simulink model "MinSeg_sim_LQR"  (R2024b)
settings: Solver=ode4  StartTime=0.0  StopTime=4  FixedStep=0.0001  RelTol=1e-3
values from neighbouring files (symbols this model uses):
  c = 0.5    [parameters.m]
  d = 0.5    [parameters.m]
  eta = 0.9    [parameters.m]
  g = 9.81    [parameters.m]
  I = M/12*(t^2 + b^2) + M*l^2    (= 0.00128463833333)    [parameters.m]
  J = 1/2*m*r^2    (= 2.7104e-05)    [parameters.m]
  K = lqr(sys_MS, Q_lqr, R_lqr)    [main.m]
  Km = 0.05    [parameters.m]
  L = 2.6e-3    (= 0.0026)    [parameters.m]    (also in pole_placement_Luenberger.m = place(A', C', desired_poles)')
  l = 0.06    [parameters.m]
  M = 0.3303 - 2*m    (= 0.2743)    [parameters.m]
  m = 0.028    [parameters.m]
  N = 50    [parameters.m]
  R = 0.5    [parameters.m]
  r = 0.044    [parameters.m]
undefined symbols (not defined in the file or in its folder): init_dq, init_q, tau_m, tau_max, theta_ref, U_max
settings Model: Creator=albin  LastModifiedBy=albin
settings DataIOCC: ExternalInput=[t, 6, 6]  ReturnWorkspaceOutputs=off

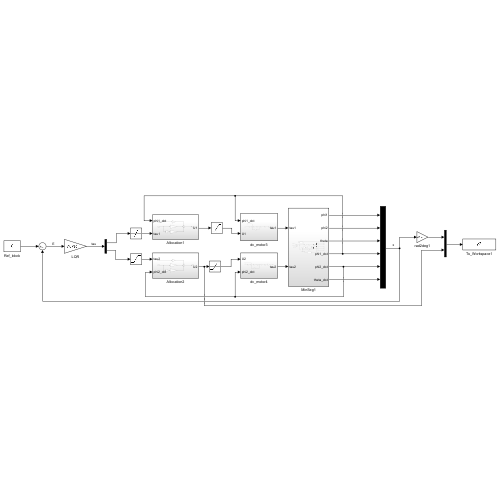
[thumbnail: Simulink's stored preview of the top-level diagram]
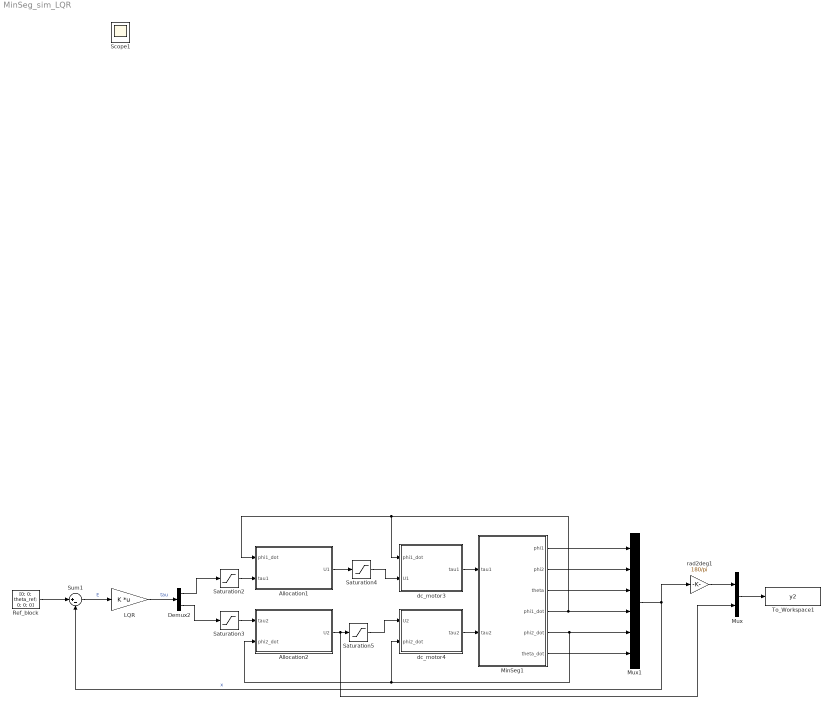
== system MinSeg_sim_LQR ==
  Allocation1 : Subsystem
  Allocation2 : Subsystem
  Demux2 : Demux  Outputs=2
  LQR : Gain  Gain=K  Multiplication=Matrix(K*u) (u vector)
  MinSeg1 : Subsystem
  Mux : Mux  Inputs=2
  Mux1 : Mux  Inputs=6
  Ref_block : Constant  Value=[0; 0; theta_ref; 0; 0; 0]
  Saturation2 : Saturate  UpperLimit=tau_max  LowerLimit=-tau_max
  Saturation3 : Saturate  UpperLimit=0.05  LowerLimit=-0.05
  Saturation4 : Saturate  UpperLimit=U_max  LowerLimit=-U_max
  Saturation5 : Saturate  UpperLimit=U_max  LowerLimit=-U_max
  Sum1 : Sum  Inputs=|+-
  To_Workspace1 : ToWorkspace  VariableName=y2  SaveFormat=Timeseries  SampleTime=-1
  dc_motor3 : Subsystem
  dc_motor4 : Subsystem
  rad2deg1 : Gain  Gain=180/pi
  Scope1 : Scope
  wires:
  Allocation2/1(U2) -> Mux/2, Saturation5/1
  dc_motor4/1(tau2) -> MinSeg1/2(tau2)
  Saturation3/1 -> Allocation2/1(tau2)
  dc_motor3/1(tau1) -> MinSeg1/1(tau1)
  LQR/1 -> Demux2/1  "tau"
  Allocation1/1(U1) -> Saturation4/1
  MinSeg1/5(phi2_dot) -> Mux1/5, dc_motor4/2(phi2_dot), Allocation2/2(phi2_dot)
  Sum1/1 -> LQR/1  "E"
  Demux2/1 -> Saturation2/1
  MinSeg1/4(phi1_dot) -> Allocation1/1(phi1_dot), dc_motor3/1(phi1_dot), Mux1/4
  Mux1/1 -> rad2deg1/1, Sum1/2  "x"
  Saturation2/1 -> Allocation1/2(tau1)
  MinSeg1/1(phi1) -> Mux1/1
  Ref_block/1 -> Sum1/1
  MinSeg1/6(theta_dot) -> Mux1/6
  MinSeg1/2(phi2) -> Mux1/2
  Saturation4/1 -> dc_motor3/2(U1)
  Saturation5/1 -> dc_motor4/1(U2)
  MinSeg1/3(theta) -> Mux1/3
  Demux2/2 -> Saturation3/1
  Mux/1 -> To_Workspace1/1
  rad2deg1/1 -> Mux/1

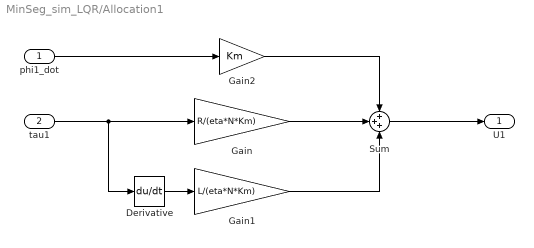
== system MinSeg_sim_LQR/Allocation1 ==
  phi1_dot : Inport
  tau1 : Inport  Port=2
  Derivative : Derivative
  Gain : Gain  Gain=R/(eta*N*Km)
  Gain1 : Gain  Gain=L/(eta*N*Km)
  Gain2 : Gain  Gain=Km
  Sum : Sum  Inputs=+++
  U1 : Outport
  wires:
  Gain1/1 -> Sum/3
  tau1/1 -> Derivative/1, Gain/1
  Gain/1 -> Sum/2
  Derivative/1 -> Gain1/1
  Sum/1 -> U1/1
  phi1_dot/1 -> Gain2/1
  Gain2/1 -> Sum/1

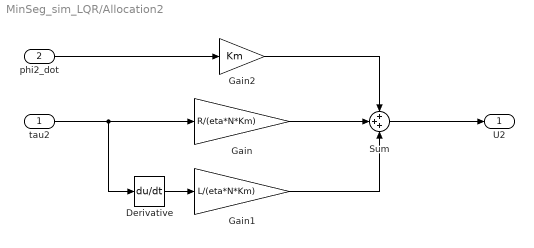
== system MinSeg_sim_LQR/Allocation2 ==
  tau2 : Inport
  phi2_dot : Inport  Port=2
  Derivative : Derivative
  Gain : Gain  Gain=R/(eta*N*Km)
  Gain1 : Gain  Gain=L/(eta*N*Km)
  Gain2 : Gain  Gain=Km
  Sum : Sum  Inputs=+++
  U2 : Outport
  wires:
  Gain1/1 -> Sum/3
  tau2/1 -> Derivative/1, Gain/1
  Gain/1 -> Sum/2
  Derivative/1 -> Gain1/1
  Sum/1 -> U2/1
  phi2_dot/1 -> Gain2/1
  Gain2/1 -> Sum/1

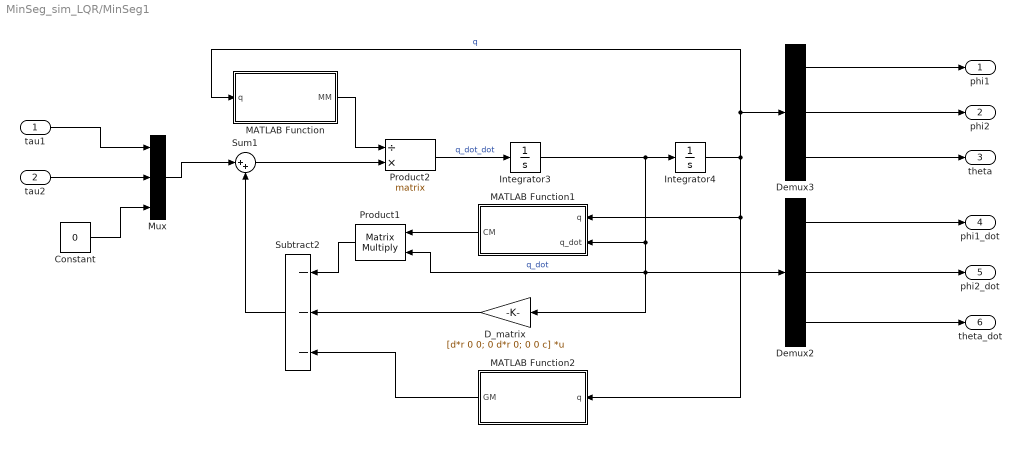
== system MinSeg_sim_LQR/MinSeg1 ==
  tau1 : Inport
  tau2 : Inport  Port=2
  Constant : Constant  Value=0
  D_matrix : Gain  Gain=[d*r 0 0; 0 d*r 0; 0 0 c]  Multiplication=Matrix(K*u)
  Demux2 : Demux  Outputs=3
  Demux3 : Demux  Outputs=3
  Integrator3 : Integrator  InitialCondition=init_dq
  Integrator4 : Integrator  InitialCondition=init_q
  MATLAB Function : MATLAB Function  TreatAsAtomicUnit=on
  MATLAB Function1 : MATLAB Function  TreatAsAtomicUnit=on
  MATLAB Function2 : MATLAB Function  TreatAsAtomicUnit=on
  Mux : Mux  Inputs=3
  Product1 : Product  Multiplication=Matrix(*)
  Product2 : Product  Inputs=/*  Multiplication=Matrix(*)
  Subtract2 : Sum  Inputs=---
  Sum1 : Sum  Inputs=|++
  phi1 : Outport
  phi2 : Outport  Port=2
  theta : Outport  Port=3
  phi1_dot : Outport  Port=4
  phi2_dot : Outport  Port=5
  theta_dot : Outport  Port=6
  wires:
  Product2/1 -> Integrator3/1  "q_dot_dot"
  Mux/1 -> Sum1/1
  Constant/1 -> Mux/3
  Integrator4/1 -> MATLAB Function2/1(q), MATLAB Function1/1(q), Demux3/1, MATLAB Function/1(q)  "q"
  Demux3/2 -> phi2/1
  Demux2/1 -> phi1_dot/1
  MATLAB Function/1(MM) -> Product2/1
  Demux3/1 -> phi1/1
  Integrator3/1 -> MATLAB Function1/2(q_dot), D_matrix/1, Product1/2, Demux2/1, Integrator4/1  "q_dot"
  MATLAB Function2/1(GM) -> Subtract2/3
  Subtract2/1 -> Sum1/2
  MATLAB Function1/1(CM) -> Product1/1
  Product1/1 -> Subtract2/1
  Demux2/3 -> theta_dot/1
  Demux2/2 -> phi2_dot/1
  Demux3/3 -> theta/1
  Sum1/1 -> Product2/2
  D_matrix/1 -> Subtract2/2
  tau1/1 -> Mux/1
  tau2/1 -> Mux/2

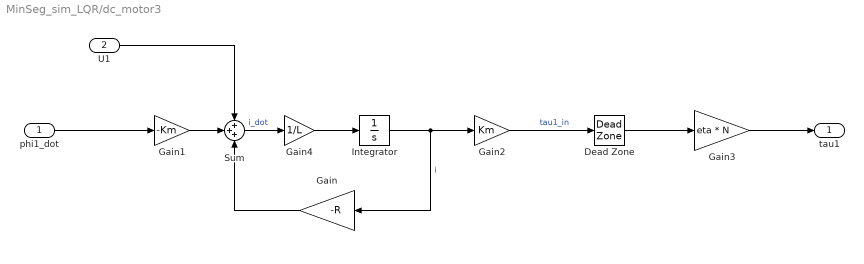
== system MinSeg_sim_LQR/dc_motor3 ==
  phi1_dot : Inport
  U1 : Inport  Port=2
  Dead Zone : DeadZone  LowerValue=-tau_m  UpperValue=tau_m
  Gain : Gain  Gain=-R
  Gain1 : Gain  Gain=-Km
  Gain2 : Gain  Gain=Km
  Gain3 : Gain  Gain=eta * N
  Gain4 : Gain  Gain=1/L
  Integrator : Integrator
  Sum : Sum  Inputs=+++
  tau1 : Outport
  wires:
  Gain2/1 -> Dead Zone/1  "tau1_in"
  Integrator/1 -> Gain/1, Gain2/1  "i"
  Gain3/1 -> tau1/1
  Gain1/1 -> Sum/2
  Gain/1 -> Sum/3
  phi1_dot/1 -> Gain1/1
  Sum/1 -> Gain4/1  "i_dot"
  Gain4/1 -> Integrator/1
  U1/1 -> Sum/1
  Dead Zone/1 -> Gain3/1

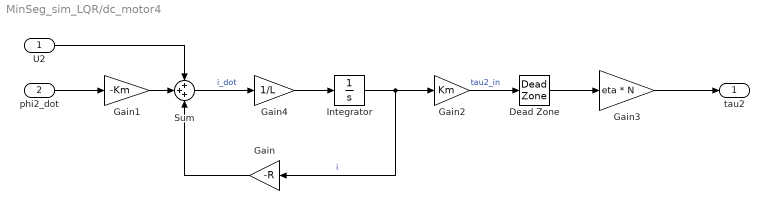
== system MinSeg_sim_LQR/dc_motor4 ==
  U2 : Inport
  phi2_dot : Inport  Port=2
  Dead Zone : DeadZone  LowerValue=-tau_m  UpperValue=tau_m
  Gain : Gain  Gain=-R
  Gain1 : Gain  Gain=-Km
  Gain2 : Gain  Gain=Km
  Gain3 : Gain  Gain=eta * N
  Gain4 : Gain  Gain=1/L
  Integrator : Integrator
  Sum : Sum  Inputs=+++
  tau2 : Outport
  wires:
  Gain2/1 -> Dead Zone/1  "tau2_in"
  Integrator/1 -> Gain/1, Gain2/1  "i"
  Gain3/1 -> tau2/1
  U2/1 -> Sum/1
  Gain1/1 -> Sum/2
  Sum/1 -> Gain4/1  "i_dot"
  phi2_dot/1 -> Gain1/1
  Gain/1 -> Sum/3
  Dead Zone/1 -> Gain3/1
  Gain4/1 -> Integrator/1

== matlab function MinSeg_sim_LQR/MinSeg1/MATLAB Function ==
  data: q input; MM output; r parameter; m parameter; M parameter; l parameter; I parameter; J parameter
function MM = M_matrix(q, r, m, M, l, I, J)
    % initialize
    MM = zeros(3,3);
    
    % extract theta from q
    theta = q(3);

    % Calculate the elements of the M(q) matrix
    MM(1,1) = r^2*(1/4*M + m) + J;
    MM(1,2) = 1/4*M*r^2;
    MM(1,3) = r^2*(1/2*M + m) + J + 1/2*M*l*r*cos(theta);
    MM(2,1) = 1/4*M*r^2;
    MM(2,2) = r^2*(1/4*M + m) + J;
    MM(2,3) = r^2*(1/2*M + m) + J + 1/2*M*l*r*cos(theta);
    MM(3,1) = r^2*(1/2*M + m) + J + 1/2*M*l*r*cos(theta);
    MM(3,2) = r^2*(1/2*M + m) + J + 1/2*M*l*r*cos(theta);
    MM(3,3) = r^2*(M + 2*m) + 2*J + 2*M*l*r*cos(theta) + M*l^2 + I;
end

== matlab function MinSeg_sim_LQR/MinSeg1/MATLAB Function1 ==
  data: q input; q_dot input; CM output; r parameter; M parameter; l parameter
function CM = C_matrix(q, q_dot, r, M, l)
    % initialize
    CM = zeros(3,3);

    % extract variables 
    theta = q(3);
    theta_dot = q_dot(3);

    % Calculate the elements of the C(q, q_dot) matrix
    CM(1,3) = -1/2*M*l*r*theta_dot*sin(theta);
    CM(2,3) = -1/2*M*l*r*theta_dot*sin(theta);
    CM(3,3) = -M*l*r*theta_dot*sin(theta);
end

== matlab function MinSeg_sim_LQR/MinSeg1/MATLAB Function2 ==
  data: q input; GM output; g parameter; M parameter; l parameter
function GM = G_matrix(q, g, M, l)
    % extract theta from q
    theta = q(3);

    % Calculate the elements of the G(q) matrix
    GM = [0; 0; -M*g*l*sin(theta)];
end
